simulink model "simpower"  (R2014b)
settings: Solver=ode15s  StartTime=0.0  StopTime=10.0  RelTol=1e-3
undefined symbols (not defined in the file or in its folder): j, pe
libraries: fl_lib x32, pe_lib x12, nesl_utility x9, simulink_extras x4
settings Model: Creator=torsteinibo  LastModifiedBy=torsteinibo

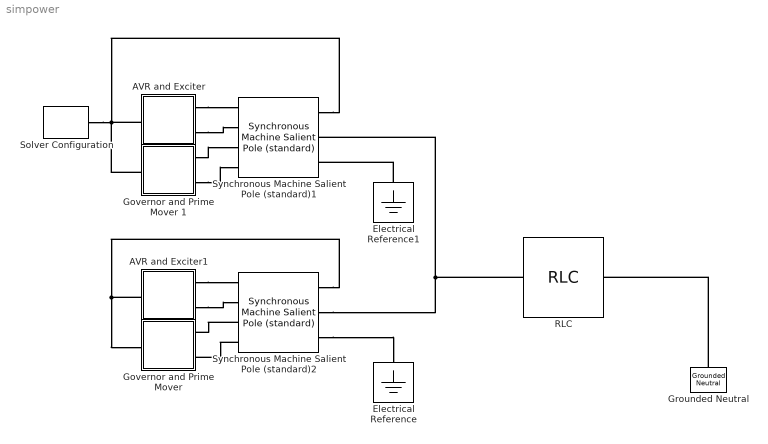
== system simpower ==
  AVR and Exciter : Subsystem
  AVR and Exciter1 : Subsystem
  Electrical Reference : fl_lib/Electrical/Electrical Elements/Electrical Reference
  Electrical Reference1 : fl_lib/Electrical/Electrical Elements/Electrical Reference
  "Governor and Prime Mover " : Subsystem  mask(Governor and Prime Mover){pu_speed_reference=0.998, droop_percentage=5, pu_load_reference_setpoint=0.5, T_G=0.2, T_CH=0.3, base_torque=1.47218e+06, pu_torque0=0.451061}
      mask prompts: pu_speed_reference "Speed reference, (pu)"; droop_percentage "Percentage droop, (%)"; pu_load_reference_setpoint "Load reference setpoint, (pu)"; T_G "Time constant of governor, (s)"; T_CH "Time constant of main inlet volumes and steam chest, (s)"; base_torque "Base torque, (N*m)"; pu_torque0 "Initial torque, (pu)"
      mask help:
      | Implements a synchronous machine governor and prime mover. The prime mover is a non-reheat steam turbine.
      |
      | The input to the block is a per-unit synchronous machine measurement vector.
      |
      | R and C are mechanical rotational ports.
  Governor and Prime Mover 1 : Subsystem  mask(Governor and Prime Mover){pu_speed_reference=0.998, droop_percentage=5, pu_load_reference_setpoint=0.5, T_G=0.2, T_CH=0.3, base_torque=1.47218e+06, pu_torque0=0.451061}
      mask prompts: pu_speed_reference "Speed reference, (pu)"; droop_percentage "Percentage droop, (%)"; pu_load_reference_setpoint "Load reference setpoint, (pu)"; T_G "Time constant of governor, (s)"; T_CH "Time constant of main inlet volumes and steam chest, (s)"; base_torque "Base torque, (N*m)"; pu_torque0 "Initial torque, (pu)"
      mask help:
      | Implements a synchronous machine governor and prime mover. The prime mover is a non-reheat steam turbine.
      |
      | The input to the block is a per-unit synchronous machine measurement vector.
      |
      | R and C are mechanical rotational ports.
  Grounded Neutral : pe_lib/Connections/Grounded Neutral
  RLC : pe_lib/Passive Devices/RLC  component_structure=1  R=1 Ohm  L=0.001 H  IL0=[ 0 0 0 ] A  C=1e-6 F  VC0=[ 0 0 0 ] V  R_parasitic=1e-6 Ohm  G_parasitic=1e-6 1/Ohm
  Solver Configuration : nesl_utility/Solver Configuration  PhysicalDomain=network_engine_domain  SubClassName=solver  LeftPortType=input  RightPortType=generic  Accelerate=off  Tones=[]  Harmonics=[]  SimulateNoise=off  Profile=off  UseLocalSampling=off  EnableSwitchedLinearOptims=on  FrequencyDomain=off  UseCCode=off  RelTol=0.001  AbsTol=1e-06  MinStep=1e-09  ToWorkspace=off  DoDC=on  ResidualTolerance=1e-09  UseLocalSolver=off  LocalSolverChoice=NE_BACKWARD_EULER_ADVANCER  LocalSolverSampleTime=1e-3  DoFixedCost=off  MaxNonlinIter=3  MaxModeIter=2  LinearAlgebra=Sparse  DelaysMemoryBudget=1024  AutomaticFiltering=on  FilteringTimeConstant=0.001
  Synchronous Machine Salient Pole (standard)1 : pe_lib/Machines/Synchronous Machine (Salient Pole)/Synchronous Machine Salient Pole (standard)  SRated=300e6 V*A  VRated=24e3 V  FRated=60 Hz  nPolePairs=10  fieldCircuitParameterization_option=2  baseEfd=216.54 V  baseIfd=1000 A  Ra=0.011  Xl=0.15  Xd=1.05  Xq=0.7  X0=0  Xdd=0.35  Xddd=0.25  Xqdd=0.325  d_transient_option=1  Td0d=5.25 s  Tdd=1.75 s  d_subtransient_option=1  Td0dd=0.03 s  Tddd=0.0214 s  q_subtransient_option=1  Tq0dd=0.05 s  Tqdd=0.0232 s  saturation_option=0  saturation_ifd=[0.00, 0.48, 0.76, 1.38, 1.79]  saturation_Vag=[0.00, 0.43, 0.59, 0.71, 0.76]  initialization_option=2  angular_position0=0 deg  pu_psid0=0  pu_psiq0=0  pu_psi00=0  pu_psifd0=0  pu_psi1d0=0  pu_psi1q0=0  Vmag0=24e3 V  Vang0=0 deg  Pt0=270e6 V*A  Qt0=0 V*A  shift_3ph=[nan, nan, nan] rad  connection_option=int32(pe.Connection.wye)  num_q_dampers=1  oneOverOmega=nan s/rad  L0=nan  Ladu=nan  Laqu=nan  Ll=nan  Lfd=nan  Rfd=nan  L1d=nan  R1d=nan  L1q=nan  R1q=nan  Xmin=1e-9  base_v=nan V  base_i=nan A  base_torque=nan N*m  base_wMechanical=nan rad/s  base_rc_efd=nan V  base_rc_ifd=nan A  base_fd_Efd=nan V  base_fd_Ifd=nan A  saturation_psi=0  saturation_K_s=1
  Synchronous Machine Salient Pole (standard)2 : pe_lib/Machines/Synchronous Machine (Salient Pole)/Synchronous Machine Salient Pole (standard)  SRated=300e6 V*A  VRated=24e3 V  FRated=60 Hz  nPolePairs=10  fieldCircuitParameterization_option=2  baseEfd=216.54 V  baseIfd=1000 A  Ra=0.011  Xl=0.15  Xd=1.05  Xq=0.7  X0=0  Xdd=0.35  Xddd=0.25  Xqdd=0.325  d_transient_option=1  Td0d=5.25 s  Tdd=1.75 s  d_subtransient_option=1  Td0dd=0.03 s  Tddd=0.0214 s  q_subtransient_option=1  Tq0dd=0.05 s  Tqdd=0.0232 s  saturation_option=0  saturation_ifd=[0.00, 0.48, 0.76, 1.38, 1.79]  saturation_Vag=[0.00, 0.43, 0.59, 0.71, 0.76]  initialization_option=2  angular_position0=0 deg  pu_psid0=0  pu_psiq0=0  pu_psi00=0  pu_psifd0=0  pu_psi1d0=0  pu_psi1q0=0  Vmag0=24e3 V  Vang0=0 deg  Pt0=270e6 V*A  Qt0=0 V*A  shift_3ph=[nan, nan, nan] rad  connection_option=int32(pe.Connection.wye)  num_q_dampers=1  oneOverOmega=nan s/rad  L0=nan  Ladu=nan  Laqu=nan  Ll=nan  Lfd=nan  Rfd=nan  L1d=nan  R1d=nan  L1q=nan  R1q=nan  Xmin=1e-9  base_v=nan V  base_i=nan A  base_torque=nan N*m  base_wMechanical=nan rad/s  base_rc_efd=nan V  base_rc_ifd=nan A  base_fd_Efd=nan V  base_fd_Ifd=nan A  saturation_psi=0  saturation_K_s=1
  connections:
  RLC/LConn1 -- Synchronous Machine Salient Pole (standard)2/RConn2 -- Synchronous Machine Salient Pole (standard)1/RConn2
  Grounded Neutral/LConn1 -- RLC/RConn1
  Electrical Reference1/LConn1 -- Synchronous Machine Salient Pole (standard)1/RConn3
  Governor and Prime Mover 1/RConn1 -- Synchronous Machine Salient Pole (standard)1/LConn3
  Governor and Prime Mover 1/RConn2 -- Synchronous Machine Salient Pole (standard)1/LConn4
  AVR and Exciter/RConn2 -- Synchronous Machine Salient Pole (standard)1/LConn2
  AVR and Exciter/RConn1 -- Synchronous Machine Salient Pole (standard)1/LConn1
  Synchronous Machine Salient Pole (standard)1/RConn1 -- Governor and Prime Mover 1/LConn1 -- Solver Configuration/RConn1 -- AVR and Exciter/LConn1
  Synchronous Machine Salient Pole (standard)2/RConn1 -- AVR and Exciter1/LConn1 -- "Governor and Prime Mover "/LConn1
  Synchronous Machine Salient Pole (standard)2/LConn3 -- "Governor and Prime Mover "/RConn1
  AVR and Exciter1/RConn1 -- Synchronous Machine Salient Pole (standard)2/LConn1
  AVR and Exciter1/RConn2 -- Synchronous Machine Salient Pole (standard)2/LConn2
  Synchronous Machine Salient Pole (standard)2/LConn4 -- "Governor and Prime Mover "/RConn2
  Synchronous Machine Salient Pole (standard)2/RConn3 -- Electrical Reference/LConn1

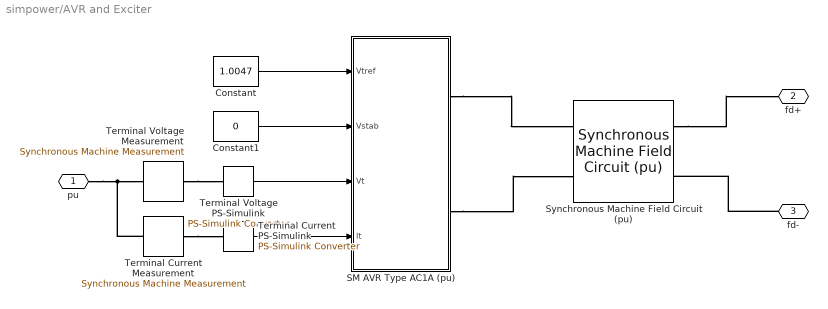
== system simpower/AVR and Exciter ==
  Constant : Constant  Value=1.0047
  Constant1 : Constant  Value=0
  SM AVR Type AC1A (pu) : Subsystem  mask(AVR and Excitation System){RcXc=[0 0], Tr=20e-3, KaTa=[400 0.02], KeTe=[1 0.8], TbTc=[0 0], KfTf=[0.03 1], Ve21=[3.14 4.18], SeVe21=[0.03 0.1], Vaminmax=[-14.5 14.5], Vrminmax=[-5.43 6.03], Kc=0.2, Kd=0.38, v0=[1.0047,1.32943]}
      mask prompts: RcXc "Compensation resistance and reactance, [Rc(pu)  Xc(pu)]:"; Tr "Voltage sensing and compensation time constant, Tr(s):"; KaTa "Voltage regulator gain and time constant, [Ka Ta(s)]:"; KeTe "Exciter field gain and time constant, [Ke Te(s)]:"; TbTc "Transient gain reduction lag and lead time constants, [Tb(s) Tc(s)]:"; KfTf "Damping filter gain and time constant, [Kf  Tf(s)]:"; Ve21 "Field voltage values, [Ve2(pu) Ve1(pu)]:"; SeVe21 "Saturation values, [SeVe2(pu) SeVe1(pu)]:"; Vaminmax "Regulator internal voltage limits, [Vamin(pu) Vamax(pu)]:"; Vrminmax "Voltage regulator output limits, [Vrmin(pu) Vrmax(pu)]:"; Kc "Rectifier regulation factor, Kc(pu):"; Kd "Exciter internal reactance, Kd(pu):"; v0 "Initial terminal voltage and initial field voltage, [Vt0(pu) Efd0(pu)]:"
      mask help:
      | Implements an AC1A synchronous machine Automatic Voltage Regulator (AVR) combined with an exciter.
      |
      | The inputs to the block are per-unit voltages and current.
      |
      | The output of the block is the per-unit field voltage (Efd(pu)).
      mask init:
      | Rc=RcXc(1);Xc=RcXc(2);
      | Ka=KaTa(1);Ta=KaTa(2);
      | Ke=KeTe(1);Te=KeTe(2);
      | Tb=TbTc(1);Tc=TbTc(2);
      | Vamin=Vaminmax(1);Vamax=Vaminmax(2);
      | Vrmin=Vrminmax(1);Vrmax=Vrminmax(2);
      | Kf=KfTf(1);Tf=KfTf(2);
      | Ve2=Ve21(1);Ve1=Ve21(2);
      | SeVe2=SeVe21(1);SeVe1=SeVe21(2);
      | Vt0=v0(1);Efd0=v0(2);
      | 
      | % initialisation
      | x0_exc=Efd0*(1+Kc*0.577);
      | 
      | Vfe0 = interp1( [0 Ve2 Ve1], [0 SeVe2 SeVe1], x0_exc )...
      |     + Ke*x0_exc...
      |     + Kd*Efd0;
      | 
      | gap = 1e-1;
      | Fex_xData = 0:gap:1+gap;
      | 
      | mode1Idx = Fex_xData <= 0.433;
      | mode2Idx = (0.433 < Fex_xData) & (Fex_xData < 0.75);
      | mode3Idx = (0.75 <= Fex_xData) & (Fex_xData <= 1);
      | mode4Idx = 1 < Fex_xData;
      | 
      | Fex_yData = zeros( size( Fex_xData ) );
      | Fex_yData( mode1Idx ) = 1 - 0.577.*Fex_xData( mode1Idx );
      | Fex_yData( mode2Idx ) = sqrt( 0.75 - Fex_xData( mode2Idx ).^2 );
      | Fex_yData( mode3Idx ) = 1.732*( 1 - Fex_xData( mode3Idx ) );
      | Fex_yData( mode4Idx ) = 0;
      | 
      | clear( 'gap', 'mode1Idx', 'mode2Idx',  'mode3Idx',  'mode4Idx' );
  Synchronous Machine Field Circuit (pu) : pe_lib/Machines/Synchronous Machine Field Circuit (pu)  SRated=555e6 V*A  FRated=60 Hz  fieldCircuitParameterization_option=2  baseEfd=92.95 V  baseIfd=1300 A  parameterization_option=2  Ladu=1.66  Rfd=0.0006  Xl=0.15  Xd=1.81  Xdd=0.3  d_transient_option=1  Td0d=8 s  Tdd=1.3260 s
  Terminal Current Measurement : pe_lib/Machines/Synchronous Machine Measurement  output_idx=15
  Terminal Current PS-Simulink : nesl_utility/PS-Simulink Converter  PhysicalDomain=network_engine_domain  SubClassName=ps_output  LeftPortType=input  RightPortType=output  PseudoPeriodic=off  Frequencies=[]  Unit=1  AffineConversion=off
  Terminal Voltage Measurement : pe_lib/Machines/Synchronous Machine Measurement  output_idx=14
  Terminal Voltage PS-Simulink : nesl_utility/PS-Simulink Converter  PhysicalDomain=network_engine_domain  SubClassName=ps_output  LeftPortType=input  RightPortType=output  PseudoPeriodic=off  Frequencies=[]  Unit=1  AffineConversion=off
  pu : PMIOPort  Port=1  Side=Left
  fd+ : PMIOPort  Port=2  Side=Right
  fd- : PMIOPort  Port=3  Side=Right
  wires:
  Constant/1 -> SM AVR Type AC1A (pu)/1(Vtref)
  Constant1/1 -> SM AVR Type AC1A (pu)/2(Vstab)
  Terminal Voltage PS-Simulink/1 -> SM AVR Type AC1A (pu)/3(Vt)
  Terminal Current PS-Simulink/1 -> SM AVR Type AC1A (pu)/4(It)
  connections:
  Terminal Current Measurement/RConn1 -- Terminal Current PS-Simulink/LConn1
  Terminal Voltage Measurement/RConn1 -- Terminal Voltage PS-Simulink/LConn1
  pu/RConn1 -- Terminal Current Measurement/LConn1 -- Terminal Voltage Measurement/LConn1
  SM AVR Type AC1A (pu)/RConn1 -- Synchronous Machine Field Circuit (pu)/LConn1
  SM AVR Type AC1A (pu)/RConn2 -- Synchronous Machine Field Circuit (pu)/LConn2
  Synchronous Machine Field Circuit (pu)/RConn1 -- fd+/RConn1
  fd-/RConn1 -- Synchronous Machine Field Circuit (pu)/RConn2

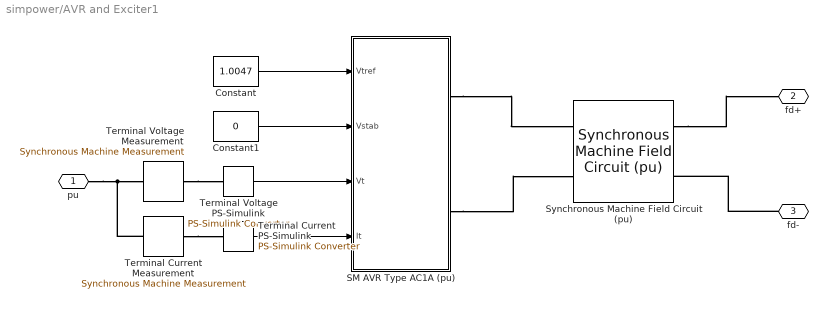
== system simpower/AVR and Exciter1 ==
  Constant : Constant  Value=1.0047
  Constant1 : Constant  Value=0
  SM AVR Type AC1A (pu) : Subsystem  mask(AVR and Excitation System){RcXc=[0 0], Tr=20e-3, KaTa=[400 0.02], KeTe=[1 0.8], TbTc=[0 0], KfTf=[0.03 1], Ve21=[3.14 4.18], SeVe21=[0.03 0.1], Vaminmax=[-14.5 14.5], Vrminmax=[-5.43 6.03], Kc=0.2, Kd=0.38, v0=[1.0047,1.32943]}
      mask prompts: RcXc "Compensation resistance and reactance, [Rc(pu)  Xc(pu)]:"; Tr "Voltage sensing and compensation time constant, Tr(s):"; KaTa "Voltage regulator gain and time constant, [Ka Ta(s)]:"; KeTe "Exciter field gain and time constant, [Ke Te(s)]:"; TbTc "Transient gain reduction lag and lead time constants, [Tb(s) Tc(s)]:"; KfTf "Damping filter gain and time constant, [Kf  Tf(s)]:"; Ve21 "Field voltage values, [Ve2(pu) Ve1(pu)]:"; SeVe21 "Saturation values, [SeVe2(pu) SeVe1(pu)]:"; Vaminmax "Regulator internal voltage limits, [Vamin(pu) Vamax(pu)]:"; Vrminmax "Voltage regulator output limits, [Vrmin(pu) Vrmax(pu)]:"; Kc "Rectifier regulation factor, Kc(pu):"; Kd "Exciter internal reactance, Kd(pu):"; v0 "Initial terminal voltage and initial field voltage, [Vt0(pu) Efd0(pu)]:"
      mask help:
      | Implements an AC1A synchronous machine Automatic Voltage Regulator (AVR) combined with an exciter.
      |
      | The inputs to the block are per-unit voltages and current.
      |
      | The output of the block is the per-unit field voltage (Efd(pu)).
      mask init: same as simpower/AVR and Exciter/SM AVR Type AC1A (pu)
  Synchronous Machine Field Circuit (pu) : pe_lib/Machines/Synchronous Machine Field Circuit (pu)  SRated=555e6 V*A  FRated=60 Hz  fieldCircuitParameterization_option=2  baseEfd=92.95 V  baseIfd=1300 A  parameterization_option=2  Ladu=1.66  Rfd=0.0006  Xl=0.15  Xd=1.81  Xdd=0.3  d_transient_option=1  Td0d=8 s  Tdd=1.3260 s
  Terminal Current Measurement : pe_lib/Machines/Synchronous Machine Measurement  output_idx=15
  Terminal Current PS-Simulink : nesl_utility/PS-Simulink Converter  PhysicalDomain=network_engine_domain  SubClassName=ps_output  LeftPortType=input  RightPortType=output  PseudoPeriodic=off  Frequencies=[]  Unit=1  AffineConversion=off
  Terminal Voltage Measurement : pe_lib/Machines/Synchronous Machine Measurement  output_idx=14
  Terminal Voltage PS-Simulink : nesl_utility/PS-Simulink Converter  PhysicalDomain=network_engine_domain  SubClassName=ps_output  LeftPortType=input  RightPortType=output  PseudoPeriodic=off  Frequencies=[]  Unit=1  AffineConversion=off
  pu : PMIOPort  Port=1  Side=Left
  fd+ : PMIOPort  Port=2  Side=Right
  fd- : PMIOPort  Port=3  Side=Right
  wires:
  Constant/1 -> SM AVR Type AC1A (pu)/1(Vtref)
  Constant1/1 -> SM AVR Type AC1A (pu)/2(Vstab)
  Terminal Voltage PS-Simulink/1 -> SM AVR Type AC1A (pu)/3(Vt)
  Terminal Current PS-Simulink/1 -> SM AVR Type AC1A (pu)/4(It)
  connections:
  Terminal Current Measurement/RConn1 -- Terminal Current PS-Simulink/LConn1
  Terminal Voltage Measurement/RConn1 -- Terminal Voltage PS-Simulink/LConn1
  pu/RConn1 -- Terminal Current Measurement/LConn1 -- Terminal Voltage Measurement/LConn1
  SM AVR Type AC1A (pu)/RConn1 -- Synchronous Machine Field Circuit (pu)/LConn1
  SM AVR Type AC1A (pu)/RConn2 -- Synchronous Machine Field Circuit (pu)/LConn2
  Synchronous Machine Field Circuit (pu)/RConn1 -- fd+/RConn1
  fd-/RConn1 -- Synchronous Machine Field Circuit (pu)/RConn2

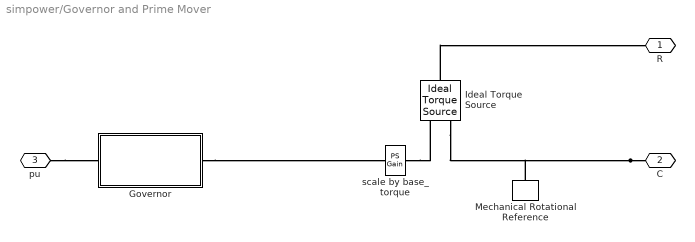
== system simpower/Governor and Prime Mover  ==
  Governor : Subsystem
  Ideal Torque Source : fl_lib/Mechanical/Mechanical Sources/Ideal Torque Source
  Mechanical Rotational Reference : fl_lib/Mechanical/Rotational Elements/Mechanical Rotational Reference
  scale by base_torque : fl_lib/Physical Signals/Functions/PS Gain  gain=base_torque
  R : PMIOPort  Port=1  Side=Right
  C : PMIOPort  Port=2  Side=Right
  pu : PMIOPort  Port=3  Side=Left
  connections:
  C/RConn1 -- Ideal Torque Source/RConn2 -- Mechanical Rotational Reference/LConn1
  Ideal Torque Source/LConn1 -- R/RConn1
  pu/RConn1 -- Governor/LConn1
  scale by base_torque/RConn1 -- Ideal Torque Source/RConn1
  Governor/RConn1 -- scale by base_torque/LConn1

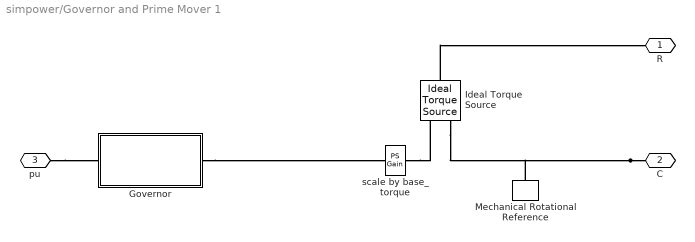
== system simpower/Governor and Prime Mover 1 ==
  Governor : Subsystem
  Ideal Torque Source : fl_lib/Mechanical/Mechanical Sources/Ideal Torque Source
  Mechanical Rotational Reference : fl_lib/Mechanical/Rotational Elements/Mechanical Rotational Reference
  scale by base_torque : fl_lib/Physical Signals/Functions/PS Gain  gain=base_torque
  R : PMIOPort  Port=1  Side=Right
  C : PMIOPort  Port=2  Side=Right
  pu : PMIOPort  Port=3  Side=Left
  connections:
  C/RConn1 -- Ideal Torque Source/RConn2 -- Mechanical Rotational Reference/LConn1
  Ideal Torque Source/LConn1 -- R/RConn1
  pu/RConn1 -- Governor/LConn1
  scale by base_torque/RConn1 -- Ideal Torque Source/RConn1
  Governor/RConn1 -- scale by base_torque/LConn1

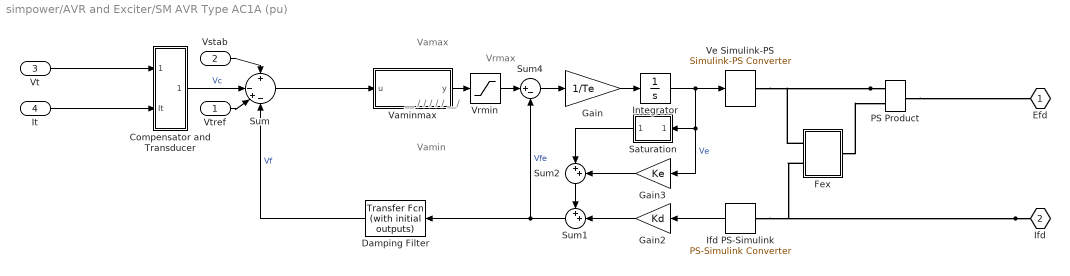
== system simpower/AVR and Exciter/SM AVR Type AC1A (pu) ==
  note: Vrmax
  note: Vamax
  note: Vamin
  note: __
      |               /
      |             /
      |           /
      |         /
      |       /
      | __/
  Vtref : Inport
  Vstab : Inport  Port=2
  Vt : Inport  Port=3
  It : Inport  Port=4
  Compensator and Transducer : Subsystem  mask{RcXc=[Rc Xc], Tr=Tr}
      mask prompts: RcXc "Compensation resistance and reactance, [Rc(pu)  Xc(pu)]:"; Tr "Voltage sensing and compensation time constant, Tr(s):"
      mask init:
      | Rc=RcXc(1);Xc=RcXc(2);
  Damping Filter : simulink_extras/Additional Linear/Transfer Fcn (with initial outputs)  N=[Kf 0]  D=[Tf 1]  Y0=-Vfe0/Ka  U0=Vfe0
  Fex : Subsystem  mask{Kc=Kc}
      mask prompts: Kc "Rectifier regulation factor, Kc(pu):"
  Gain : Gain  Gain=1/Te  SaturateOnIntegerOverflow=on  OutDataTypeStr=Inherit: Same as input  ParamDataTypeStr=Inherit: Same as input
  Gain2 : Gain  Gain=Kd  SaturateOnIntegerOverflow=on  OutDataTypeStr=Inherit: Same as input  ParamDataTypeStr=Inherit: Same as input
  Gain3 : Gain  Gain=Ke  SaturateOnIntegerOverflow=on  OutDataTypeStr=Inherit: Same as input  ParamDataTypeStr=Inherit: Same as input
  Ifd PS-Simulink : nesl_utility/PS-Simulink Converter  PhysicalDomain=network_engine_domain  SubClassName=ps_output  LeftPortType=input  RightPortType=output  PseudoPeriodic=off  Frequencies=[]  Unit=1  AffineConversion=off
  Integrator : Integrator  InitialCondition=x0_exc  LimitOutput=on  LowerSaturationLimit=0
  PS Product : fl_lib/Physical Signals/Functions/PS Product
  Saturation : Subsystem  mask{Ve21=[Ve2 Ve1], SeVe21=[SeVe2 SeVe1]}
      mask prompts: Ve21 "Field voltage values, [Ve2(pu) Ve1(pu)]:"; SeVe21 "Saturation values, [SeVe2(pu) SeVe1(pu)]:"
      mask init:
      | Ve2=Ve21(1);Ve1=Ve21(2);
      | SeVe2=SeVe21(1);SeVe1=SeVe21(2);
  Sum : Sum  Inputs=+|-+-  SaturateOnIntegerOverflow=on  InputSameDT=on  OutDataTypeStr=Inherit: Same as first input
  Sum1 : Sum  Inputs=++|  SaturateOnIntegerOverflow=on  InputSameDT=on  OutDataTypeStr=Inherit: Same as first input
  Sum2 : Sum  Inputs=|++  SaturateOnIntegerOverflow=on  InputSameDT=on  OutDataTypeStr=Inherit: Same as first input
  Sum4 : Sum  Inputs=|+-  SaturateOnIntegerOverflow=on  InputSameDT=on  OutDataTypeStr=Inherit: Same as first input
  Vaminmax : Subsystem  mask{Ka=Ka, Ta=Ta, Vaminmax=[Vamin Vamax], X0=Vfe0}
      mask prompts: Ka "Voltage regulator gain, Ka"; Ta "Voltage regulator time constant, Ta(s)"; Vaminmax "Regulator internal voltage limits, [Vamin(pu) Vamax(pu)]:"; X0 "Initial conditions:"
      mask init:
      | Vamin=Vaminmax(1);Vamax=Vaminmax(2);
      mask Display: dpoly([Ka],[Ta 1],'s')
  "Ve Simulink-PS " : nesl_utility/Simulink-PS Converter  PhysicalDomain=network_engine_domain  SubClassName=ps_input  LeftPortType=input  RightPortType=output  PseudoPeriodic=off  Frequencies=[]  NoiseDistribution=none  NoiseParameters=[]  Unit=1  AffineConversion=off  InputFiltering=off  SimscapeFilterOrder=1  InputFilterTimeConstant=.001  UdotUserProvided=[]
  Vrmin : Saturate  UpperLimit=Vrmax  LowerLimit=Vrmin
  Efd : PMIOPort  Port=1  Side=Right
  Ifd : PMIOPort  Port=2  Side=Right
  wires:
  Ifd PS-Simulink/1 -> Gain2/1
  Vt/1 -> Compensator and Transducer/1(Vt)
  Vtref/1 -> Sum/3
  Vstab/1 -> Sum/1
  Damping Filter/1 -> Sum/4  "Vf"
  Vrmin/1 -> Sum4/1
  Sum1/1 -> Sum4/2, Damping Filter/1  "Vfe"
  Gain/1 -> Integrator/1
  Integrator/1 -> Saturation/1(Ve), Gain3/1, "Ve Simulink-PS "/1  "Ve"
  Sum2/1 -> Sum1/1
  Gain2/1 -> Sum1/2
  Gain3/1 -> Sum2/2
  Saturation/1(Vx) -> Sum2/1
  It/1 -> Compensator and Transducer/2(It)
  Sum4/1 -> Gain/1
  Vaminmax/1(y) -> Vrmin/1
  Sum/1 -> Vaminmax/1(u)
  Compensator and Transducer/1(Vc) -> Sum/2  "Vc"
  connections:
  Ifd/RConn1 -- Fex/LConn2 -- Ifd PS-Simulink/LConn1
  PS Product/RConn1 -- Efd/RConn1
  PS Product/LConn1 -- Fex/LConn1 -- "Ve Simulink-PS "/RConn1
  Fex/RConn1 -- PS Product/LConn2

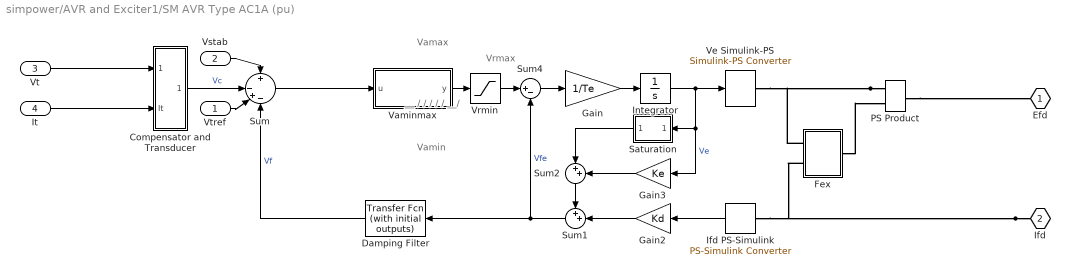
== system simpower/AVR and Exciter1/SM AVR Type AC1A (pu) ==
  note: Vrmax
  note: Vamax
  note: Vamin
  note: __
      |               /
      |             /
      |           /
      |         /
      |       /
      | __/
  Vtref : Inport
  Vstab : Inport  Port=2
  Vt : Inport  Port=3
  It : Inport  Port=4
  Compensator and Transducer : Subsystem  mask{RcXc=[Rc Xc], Tr=Tr}
      mask prompts: RcXc "Compensation resistance and reactance, [Rc(pu)  Xc(pu)]:"; Tr "Voltage sensing and compensation time constant, Tr(s):"
      mask init:
      | Rc=RcXc(1);Xc=RcXc(2);
  Damping Filter : simulink_extras/Additional Linear/Transfer Fcn (with initial outputs)  N=[Kf 0]  D=[Tf 1]  Y0=-Vfe0/Ka  U0=Vfe0
  Fex : Subsystem  mask{Kc=Kc}
      mask prompts: Kc "Rectifier regulation factor, Kc(pu):"
  Gain : Gain  Gain=1/Te  SaturateOnIntegerOverflow=on  OutDataTypeStr=Inherit: Same as input  ParamDataTypeStr=Inherit: Same as input
  Gain2 : Gain  Gain=Kd  SaturateOnIntegerOverflow=on  OutDataTypeStr=Inherit: Same as input  ParamDataTypeStr=Inherit: Same as input
  Gain3 : Gain  Gain=Ke  SaturateOnIntegerOverflow=on  OutDataTypeStr=Inherit: Same as input  ParamDataTypeStr=Inherit: Same as input
  Ifd PS-Simulink : nesl_utility/PS-Simulink Converter  PhysicalDomain=network_engine_domain  SubClassName=ps_output  LeftPortType=input  RightPortType=output  PseudoPeriodic=off  Frequencies=[]  Unit=1  AffineConversion=off
  Integrator : Integrator  InitialCondition=x0_exc  LimitOutput=on  LowerSaturationLimit=0
  PS Product : fl_lib/Physical Signals/Functions/PS Product
  Saturation : Subsystem  mask{Ve21=[Ve2 Ve1], SeVe21=[SeVe2 SeVe1]}
      mask prompts: Ve21 "Field voltage values, [Ve2(pu) Ve1(pu)]:"; SeVe21 "Saturation values, [SeVe2(pu) SeVe1(pu)]:"
      mask init:
      | Ve2=Ve21(1);Ve1=Ve21(2);
      | SeVe2=SeVe21(1);SeVe1=SeVe21(2);
  Sum : Sum  Inputs=+|-+-  SaturateOnIntegerOverflow=on  InputSameDT=on  OutDataTypeStr=Inherit: Same as first input
  Sum1 : Sum  Inputs=++|  SaturateOnIntegerOverflow=on  InputSameDT=on  OutDataTypeStr=Inherit: Same as first input
  Sum2 : Sum  Inputs=|++  SaturateOnIntegerOverflow=on  InputSameDT=on  OutDataTypeStr=Inherit: Same as first input
  Sum4 : Sum  Inputs=|+-  SaturateOnIntegerOverflow=on  InputSameDT=on  OutDataTypeStr=Inherit: Same as first input
  Vaminmax : Subsystem  mask{Ka=Ka, Ta=Ta, Vaminmax=[Vamin Vamax], X0=Vfe0}
      mask prompts: Ka "Voltage regulator gain, Ka"; Ta "Voltage regulator time constant, Ta(s)"; Vaminmax "Regulator internal voltage limits, [Vamin(pu) Vamax(pu)]:"; X0 "Initial conditions:"
      mask init:
      | Vamin=Vaminmax(1);Vamax=Vaminmax(2);
      mask Display: dpoly([Ka],[Ta 1],'s')
  "Ve Simulink-PS " : nesl_utility/Simulink-PS Converter  PhysicalDomain=network_engine_domain  SubClassName=ps_input  LeftPortType=input  RightPortType=output  PseudoPeriodic=off  Frequencies=[]  NoiseDistribution=none  NoiseParameters=[]  Unit=1  AffineConversion=off  InputFiltering=off  SimscapeFilterOrder=1  InputFilterTimeConstant=.001  UdotUserProvided=[]
  Vrmin : Saturate  UpperLimit=Vrmax  LowerLimit=Vrmin
  Efd : PMIOPort  Port=1  Side=Right
  Ifd : PMIOPort  Port=2  Side=Right
  wires:
  Ifd PS-Simulink/1 -> Gain2/1
  Vt/1 -> Compensator and Transducer/1(Vt)
  Vtref/1 -> Sum/3
  Vstab/1 -> Sum/1
  Damping Filter/1 -> Sum/4  "Vf"
  Vrmin/1 -> Sum4/1
  Sum1/1 -> Sum4/2, Damping Filter/1  "Vfe"
  Gain/1 -> Integrator/1
  Integrator/1 -> Saturation/1(Ve), Gain3/1, "Ve Simulink-PS "/1  "Ve"
  Sum2/1 -> Sum1/1
  Gain2/1 -> Sum1/2
  Gain3/1 -> Sum2/2
  Saturation/1(Vx) -> Sum2/1
  It/1 -> Compensator and Transducer/2(It)
  Sum4/1 -> Gain/1
  Vaminmax/1(y) -> Vrmin/1
  Sum/1 -> Vaminmax/1(u)
  Compensator and Transducer/1(Vc) -> Sum/2  "Vc"
  connections:
  Ifd/RConn1 -- Fex/LConn2 -- Ifd PS-Simulink/LConn1
  PS Product/RConn1 -- Efd/RConn1
  PS Product/LConn1 -- Fex/LConn1 -- "Ve Simulink-PS "/RConn1
  Fex/RConn1 -- PS Product/LConn2

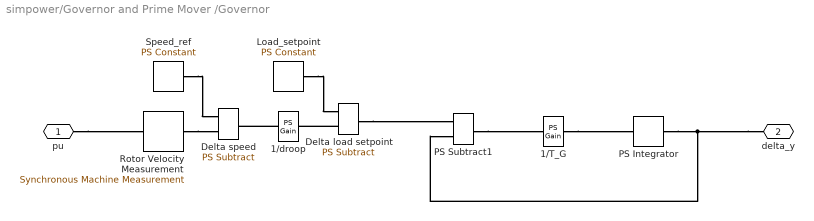
== system simpower/Governor and Prime Mover /Governor ==
  1/T_G : fl_lib/Physical Signals/Functions/PS Gain  gain=1/T_G
  1/droop : fl_lib/Physical Signals/Functions/PS Gain  gain=1/(droop_percentage/100)
  Delta load setpoint : fl_lib/Physical Signals/Functions/PS Subtract
  Delta speed : fl_lib/Physical Signals/Functions/PS Subtract
  Load_setpoint : fl_lib/Physical Signals/Sources/PS Constant  constant=pu_load_reference_setpoint
  PS Integrator : fl_lib/Physical Signals/Linear Operators/PS Integrator  x0=pu_torque0
  PS Subtract1 : fl_lib/Physical Signals/Functions/PS Subtract
  Rotor Velocity Measurement : pe_lib/Machines/Synchronous Machine Measurement  output_idx=4
  Speed_ref : fl_lib/Physical Signals/Sources/PS Constant  constant=pu_speed_reference
  pu : PMIOPort  Port=1  Side=Left
  delta_y : PMIOPort  Port=2  Side=Right
  connections:
  delta_y/RConn1 -- PS Subtract1/LConn2 -- PS Integrator/RConn1
  PS Subtract1/RConn1 -- 1/T_G/LConn1
  1/T_G/RConn1 -- PS Integrator/LConn1
  Load_setpoint/RConn1 -- Delta load setpoint/LConn1
  1/droop/LConn1 -- Delta speed/RConn1
  Speed_ref/RConn1 -- Delta speed/LConn2
  Rotor Velocity Measurement/RConn1 -- Delta speed/LConn1
  Delta load setpoint/LConn2 -- 1/droop/RConn1
  Delta load setpoint/RConn1 -- PS Subtract1/LConn1
  pu/RConn1 -- Rotor Velocity Measurement/LConn1

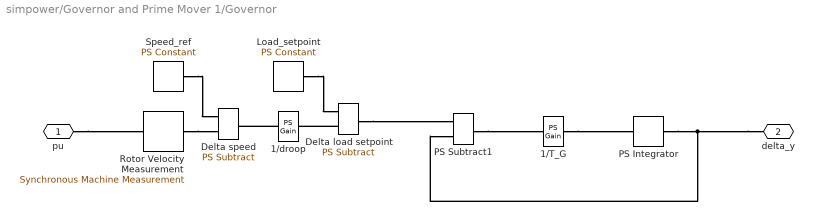
== system simpower/Governor and Prime Mover 1/Governor ==
  1/T_G : fl_lib/Physical Signals/Functions/PS Gain  gain=1/T_G
  1/droop : fl_lib/Physical Signals/Functions/PS Gain  gain=1/(droop_percentage/100)
  Delta load setpoint : fl_lib/Physical Signals/Functions/PS Subtract
  Delta speed : fl_lib/Physical Signals/Functions/PS Subtract
  Load_setpoint : fl_lib/Physical Signals/Sources/PS Constant  constant=pu_load_reference_setpoint
  PS Integrator : fl_lib/Physical Signals/Linear Operators/PS Integrator  x0=pu_torque0
  PS Subtract1 : fl_lib/Physical Signals/Functions/PS Subtract
  Rotor Velocity Measurement : pe_lib/Machines/Synchronous Machine Measurement  output_idx=4
  Speed_ref : fl_lib/Physical Signals/Sources/PS Constant  constant=pu_speed_reference
  pu : PMIOPort  Port=1  Side=Left
  delta_y : PMIOPort  Port=2  Side=Right
  connections:
  delta_y/RConn1 -- PS Subtract1/LConn2 -- PS Integrator/RConn1
  PS Subtract1/RConn1 -- 1/T_G/LConn1
  1/T_G/RConn1 -- PS Integrator/LConn1
  Load_setpoint/RConn1 -- Delta load setpoint/LConn1
  1/droop/LConn1 -- Delta speed/RConn1
  Speed_ref/RConn1 -- Delta speed/LConn2
  Rotor Velocity Measurement/RConn1 -- Delta speed/LConn1
  Delta load setpoint/LConn2 -- 1/droop/RConn1
  Delta load setpoint/RConn1 -- PS Subtract1/LConn1
  pu/RConn1 -- Rotor Velocity Measurement/LConn1

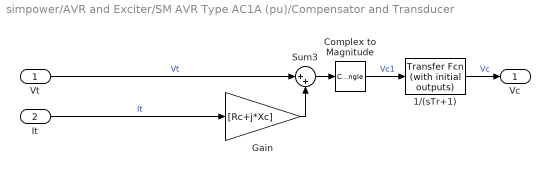
== system simpower/AVR and Exciter/SM AVR Type AC1A (pu)/Compensator and Transducer ==
  Vt : Inport
  It : Inport  Port=2
  1/(sTr+1) : simulink_extras/Additional Linear/Transfer Fcn (with initial outputs)  N=1  D=[Tr 1]  Y0=Vt0  U0=Vt0
  Complex to Magnitude : ComplexToMagnitudeAngle  Output=Magnitude
  Gain : Gain  Gain=[Rc+j*Xc]  SaturateOnIntegerOverflow=on  OutDataTypeStr=Inherit: Same as input  ParamDataTypeStr=Inherit: Same as input
  Sum3 : Sum  Inputs=|++  SaturateOnIntegerOverflow=on  InputSameDT=on  OutDataTypeStr=Inherit: Same as first input
  Vc : Outport
  wires:
  Vt/1 -> Sum3/1  "Vt"
  It/1 -> Gain/1  "It"
  Gain/1 -> Sum3/2
  Sum3/1 -> Complex to Magnitude/1
  Complex to Magnitude/1 -> 1/(sTr+1)/1  "Vc1"
  1/(sTr+1)/1 -> Vc/1  "Vc"

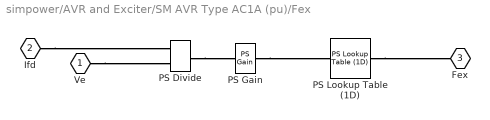
== system simpower/AVR and Exciter/SM AVR Type AC1A (pu)/Fex ==
  PS Divide : fl_lib/Physical Signals/Functions/PS Divide
  PS Gain : fl_lib/Physical Signals/Functions/PS Gain  gain=Kc
  PS Lookup Table (1D) : fl_lib/Physical Signals/Lookup Tables/PS Lookup Table (1D)  x_t=Fex_xData  y_t=Fex_yData  interp_method=1  extrap_method=1
  Ve : PMIOPort  Port=1  Side=Left
  Ifd : PMIOPort  Port=2  Side=Left
  Fex : PMIOPort  Port=3  Side=Right
  connections:
  PS Lookup Table (1D)/RConn1 -- Fex/RConn1
  PS Gain/RConn1 -- PS Lookup Table (1D)/LConn1
  PS Divide/RConn1 -- PS Gain/LConn1
  Ve/RConn1 -- PS Divide/LConn2
  Ifd/RConn1 -- PS Divide/LConn1

== system simpower/AVR and Exciter/SM AVR Type AC1A (pu)/Saturation ==
  Ve : Inport
  Product : Product  SaturateOnIntegerOverflow=on  RndMeth=Zero  InputSameDT=on  OutDataTypeStr=Inherit: Same as first input
  Saturation : Lookup  InputValues=[0 Ve2 Ve1]  Table=[0 SeVe2 SeVe1]  SaturateOnIntegerOverflow=on
  Vx : Outport
  wires:
  Ve/1 -> Product/1, Saturation/1
  Saturation/1 -> Product/2
  Product/1 -> Vx/1

== system simpower/AVR and Exciter/SM AVR Type AC1A (pu)/Vaminmax ==
  u : Inport
  Gain1 : Gain  Gain=1/Ta  SaturateOnIntegerOverflow=on  OutDataTypeStr=Inherit: Same as input  ParamDataTypeStr=Inherit: Same as input
  Gain2 : Gain  Gain=Ka  SaturateOnIntegerOverflow=on  OutDataTypeStr=Inherit: Same as input  ParamDataTypeStr=Inherit: Same as input
  Integrator : Integrator  InitialCondition=X0  LimitOutput=on  UpperSaturationLimit=Vamax  LowerSaturationLimit=Vamin
  Sum : Sum  Inputs=|+-  SaturateOnIntegerOverflow=on  InputSameDT=on  OutDataTypeStr=Inherit: Same as first input
  y : Outport
  wires:
  u/1 -> Gain2/1
  Sum/1 -> Gain1/1
  Integrator/1 -> y/1, Sum/2
  Gain2/1 -> Sum/1
  Gain1/1 -> Integrator/1

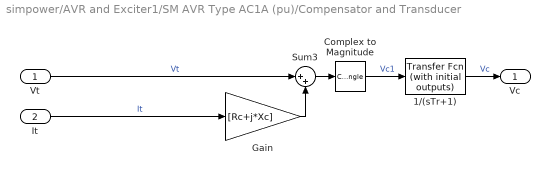
== system simpower/AVR and Exciter1/SM AVR Type AC1A (pu)/Compensator and Transducer ==
  Vt : Inport
  It : Inport  Port=2
  1/(sTr+1) : simulink_extras/Additional Linear/Transfer Fcn (with initial outputs)  N=1  D=[Tr 1]  Y0=Vt0  U0=Vt0
  Complex to Magnitude : ComplexToMagnitudeAngle  Output=Magnitude
  Gain : Gain  Gain=[Rc+j*Xc]  SaturateOnIntegerOverflow=on  OutDataTypeStr=Inherit: Same as input  ParamDataTypeStr=Inherit: Same as input
  Sum3 : Sum  Inputs=|++  SaturateOnIntegerOverflow=on  InputSameDT=on  OutDataTypeStr=Inherit: Same as first input
  Vc : Outport
  wires:
  Vt/1 -> Sum3/1  "Vt"
  It/1 -> Gain/1  "It"
  Gain/1 -> Sum3/2
  Sum3/1 -> Complex to Magnitude/1
  Complex to Magnitude/1 -> 1/(sTr+1)/1  "Vc1"
  1/(sTr+1)/1 -> Vc/1  "Vc"

== system simpower/AVR and Exciter1/SM AVR Type AC1A (pu)/Fex ==
  PS Divide : fl_lib/Physical Signals/Functions/PS Divide
  PS Gain : fl_lib/Physical Signals/Functions/PS Gain  gain=Kc
  PS Lookup Table (1D) : fl_lib/Physical Signals/Lookup Tables/PS Lookup Table (1D)  x_t=Fex_xData  y_t=Fex_yData  interp_method=1  extrap_method=1
  Ve : PMIOPort  Port=1  Side=Left
  Ifd : PMIOPort  Port=2  Side=Left
  Fex : PMIOPort  Port=3  Side=Right
  connections:
  PS Lookup Table (1D)/RConn1 -- Fex/RConn1
  PS Gain/RConn1 -- PS Lookup Table (1D)/LConn1
  PS Divide/RConn1 -- PS Gain/LConn1
  Ve/RConn1 -- PS Divide/LConn2
  Ifd/RConn1 -- PS Divide/LConn1

== system simpower/AVR and Exciter1/SM AVR Type AC1A (pu)/Saturation ==
  Ve : Inport
  Product : Product  SaturateOnIntegerOverflow=on  RndMeth=Zero  InputSameDT=on  OutDataTypeStr=Inherit: Same as first input
  Saturation : Lookup  InputValues=[0 Ve2 Ve1]  Table=[0 SeVe2 SeVe1]  SaturateOnIntegerOverflow=on
  Vx : Outport
  wires:
  Ve/1 -> Product/1, Saturation/1
  Saturation/1 -> Product/2
  Product/1 -> Vx/1

== system simpower/AVR and Exciter1/SM AVR Type AC1A (pu)/Vaminmax ==
  u : Inport
  Gain1 : Gain  Gain=1/Ta  SaturateOnIntegerOverflow=on  OutDataTypeStr=Inherit: Same as input  ParamDataTypeStr=Inherit: Same as input
  Gain2 : Gain  Gain=Ka  SaturateOnIntegerOverflow=on  OutDataTypeStr=Inherit: Same as input  ParamDataTypeStr=Inherit: Same as input
  Integrator : Integrator  InitialCondition=X0  LimitOutput=on  UpperSaturationLimit=Vamax  LowerSaturationLimit=Vamin
  Sum : Sum  Inputs=|+-  SaturateOnIntegerOverflow=on  InputSameDT=on  OutDataTypeStr=Inherit: Same as first input
  y : Outport
  wires:
  u/1 -> Gain2/1
  Sum/1 -> Gain1/1
  Integrator/1 -> y/1, Sum/2
  Gain2/1 -> Sum/1
  Gain1/1 -> Integrator/1
